simulink model "p31"  (R2021a)
settings: Solver=FixedStepDiscrete  StartTime=0.0  StopTime=5  FixedStep=1/44100  RelTol=1e-3  EnableMultiTasking=on
settings Model: SILPILModeSetting=veronly  EnablePacing=on  PacingRate=0.100000  ExtModeTrigDuration=2  Creator=Abbas  LastModifiedBy=Abbas
settings SolverCC: AutoInsertRateTranBlk=on
settings OptimizationCC: UseDivisionForNetSlopeComputation=on  GainParamInheritBuiltInType=on  UseFloatMulNetSlope=on  EnhancedBackFolding=on  PassReuseOutputArgsAs=Individual arguments  ZeroExternalMemoryAtStartup=off  ZeroInternalMemoryAtStartup=off  MaxStackSize=64  OptimizeBlockOrder=speed  DifferentSizesBufferReuse=on  OptimizationCustomize=off  EfficientTunableParamExpr=on
settings DebuggingCC: SignalRangeChecking=warning  ParameterTunabilityLossMsg=error
settings HardwareCC: ProdBitPerInt=16  ProdBitPerPointer=16  ProdBitPerSizeT=16  ProdBitPerPtrDiffT=16  ProdLargestAtomicFloat=None  ProdWordSize=8  ProdHWDeviceType=Atmel->AVR
settings SFSimCC: MATLABDynamicMemAlloc=off
settings RTWCC: SystemTargetFile=ert.tlc  HardwareBoard=Arduino Mega 2560  GenCodeOnly=on  TemplateMakefile=ert_default_tmf  GenerateReport=on  Toolchain=Arduino AVR  BuildConfiguration=Faster Runs  LaunchReport=on  GenerateWebview=on
settings CodeAppCC: ForceParamTrailComments=on  IgnoreCustomStorageClasses=off  OperatorAnnotations=on  SimulinkDataObjDesc=on  SFDataObjDesc=on  InsertBlockDesc=on
settings ERTTargetCC: SuppressErrorStatus=on  SupportNonFinite=off  SupportComplex=off  SupportContinuousTime=on  SupportVariableSizeSignals=on  ExtModeStaticAllocSize=2048

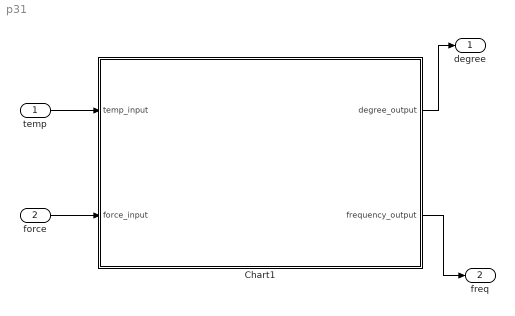
== system p31 ==
  temp : Inport  OutDataTypeStr=fixdt(1,16,4)
  force : Inport  Port=2  OutDataTypeStr=fixdt(1,16,4)
  Chart1 : Stateflow chart  TreatAsAtomicUnit=on
  degree : Outport
  freq : Outport  Port=2
  wires:
  force/1 -> Chart1/2(force_input)
  temp/1 -> Chart1/1(temp_input)
  Chart1/1(degree_output) -> degree/1
  Chart1/2(frequency_output) -> freq/1

== stateflow chart p31/Chart1 ==
  settings: updateMethod=DISCRETE  sampleTime=1
  state state2 [parallel]
    settings: executionOrder=1
    state fsr402
      entry:
    (default) -> fsr402
    fsr402 -> fsr402 [order 2] : [timerforce<2]{timerforce = timerforce+1;}
    fsr402 -> fsr402 [order 1] : [timerforce>=2]{degree_output = (force_input * 18);timerforce =0;}
  state state [parallel]
    settings: executionOrder=2
    state temp36
    (default) -> temp36
    temp36 -> temp36 [order 2] : [timertemp<1]{timertemp = timertemp+1;}
    temp36 -> temp36 [order 1] : [timertemp>=1]{frequency_output = (temp_input-20);   timertemp = 0;}
  (default) -> state2 [order 2]
  (default) -> state [order 1]
  data: temp_input input fixdt(1,16,4); force_input input fixdt(1,16,4); degree_output output fixdt(1,16,4); frequency_output output fixdt(1,16,10); timerforce local fixdt(0,16,14); timertemp local fixdt(0,16,15)
  data timerforce settings: updateMethod=SF_CONTINUOUS_TIME_DATA
  data timertemp settings: updateMethod=SF_CONTINUOUS_TIME_DATA
